simulink model "Senorless"  (R2023a)
settings: Solver=FixedStepDiscrete  StartTime=0.0  StopTime=5  FixedStep=1/FOC_FRQ  RelTol=1e-3
values from neighbouring files (symbols this model uses):
  ADC_REF = 3.6    [Senorless.sldd]
  ADC_SAMPLE_MAX = 32767.0    [Senorless.sldd]
  AMP_GAIN = 16.0    [Senorless.sldd]
  CURR_INPUT = 3276.0    [Senorless.sldd]
  CURR_KI = 380.0    [Senorless.sldd]
  CURR_KP = 0.04    [Senorless.sldd]
  CURR_LIMIT = 0.95    [Senorless.sldd]
  CURR_OVER = 6.0    [Senorless.sldd]
  CURR_POINT_GAIN = 7.0    [Senorless.sldd]
  CURR_STEP = 32760.0    [Senorless.sldd]
  CURR_UNDER = 0.03    [Senorless.sldd]
  CURR_WIDTH = 6552.0    [Senorless.sldd]
  FOC_FRQ = 25000.0    [Senorless.sldd]
  GAMMA = 32767.0    [Senorless.sldd]
  IMAX = 10.0    [Senorless.sldd]
  LPF_FRQ = 2000.0    [Senorless.sldd]
  MOTOR_DAMPER = 2.06E-7    [Senorless.sldd]
  MOTOR_FLUX = 0.00212352    [Senorless.sldd]
  MOTOR_INERTIA = 4.0E-7    [Senorless.sldd]
  MOTOR_LS = 0.000536    [Senorless.sldd]
  MOTOR_PN = 7.0    [Senorless.sldd]
  MOTOR_RS = 4.0    [Senorless.sldd]
  OPEN_IQ = 0.28    [Senorless.sldd]
  OPEN_IQ_MIN = 0.05    [Senorless.sldd]
  OPEN_IQ_SLOW = 0.1    [Senorless.sldd]
  OPEN_SPD = 1000.0    [Senorless.sldd]
  OPEN_SPD_SLOW = 180.0    [Senorless.sldd]
  OPEN_TIME = 0.5    [Senorless.sldd]
  OPEN_TIME_NFO = 0.5    [Senorless.sldd]
  PLL_LIMIT = 0.9    [Senorless.sldd]
  PLL_WIDTH = 800.0    [Senorless.sldd]
  PWM_FRQ = 96000000.0    [Senorless.sldd]
  RS_HUNT = 0.02    [Senorless.sldd]
  SMOK_FRQ = 600.0    [Senorless.sldd]
  SPD_LIMIT = 0.9    [Senorless.sldd]
  SPD_LPF_LEVEL = 0.0    [Senorless.sldd]
  SPD_MAX = 12000.0    [Senorless.sldd]
  SPD_MIN = 4000.0    [Senorless.sldd]
  SPD_REDUCE = 380.0    [Senorless.sldd]
  SPD_STEP = 6.0    [Senorless.sldd]
  SPD_WIDTH = 20.0    [Senorless.sldd]
  THETA_ERR_LIMIT = 8192.0    [Senorless.sldd]
  TS_POINT_GAIN = 10.0    [Senorless.sldd]
  UDC = 48.0    [Senorless.sldd]
  UDC_GAIN = 21.0    [Senorless.sldd]
  UDC_POINT_GAIN = 10.0    [Senorless.sldd]
undefined symbols (not defined in the file or in its folder): curr_q_ki, curr_q_kp, DiscIntNeverNeededParam, magnitude, PLL_LPF_LEVEL, Udc
libraries: simulink x20, slpidlib x5, mcbcontrolslib x2, mcbplantlib x1, autolibpmsmexterior x1, spspowerguiLib x1
(part 8 of 8)

== matlab function Senorless/FOC_PointModel/慢速开环/FreqGenerator_point2/MATLAB Function1 ==
  data: u input; y output; K_fixed input; freq_kHz input; resetTrig input; resetValue input; lowerLimit input; upperLimit input
function y = edgeTri_fixedPointIntegrator(u, K_fixed, freq_kHz, resetTrig, resetValue, lowerLimit, upperLimit)
% fixedPointIntegrator - 定点积分器（频率输入 + 复位 + 限幅 + 初始值）
%
% 输入参数说明：
%   u           - 当前输入信号（int32）
%   K_fixed     - 积分增益（已放大后的定点值，int32）
%   freq_kHz    - 控制频率（单位：kHz，如 20 表示 20kHz）
%   resetTrig   - 复位触发信号（uint8，边沿触发复位）
%   resetValue  - 复位时的初始值（int64）
%   lowerLimit  - 输出最小值（int64）
%   upperLimit  - 输出最大值（int64）
%
% 输出：
%   y           - 当前积分输出（int64）

    % 用于检测上升沿
    persistent lastResetState;
    if isempty(lastResetState)
        lastResetState = uint8(1);
    end

    % 状态变量
    persistent integratorState;
    if isempty(integratorState)
        integratorState = int64(0);
    end

    % 检测是否发生边沿触发（上升沿 或 下降沿）
    edgeTriggered = (resetTrig ~= lastResetState);

    % 如果有边沿，则复位积分器
    if edgeTriggered
        integratorState = resetValue;
    else
        % 计算 Ts（单位：μs），即 Ts = 1_000_000 / (freq_kHz * 1000)
        Ts_us = int32(1000 / freq_kHz);  % 精确到 μs（微秒）

        % 计算积分增量：delta = (K_fixed * u * Ts_us) / 1_000_000
        delta = (int64(K_fixed) * int64(u) * int64(Ts_us)) / 1000000;

        % 更新积分状态
        integratorState = integratorState + delta;

        % 饱和处理
        if integratorState > upperLimit
            integratorState = upperLimit;
        elseif integratorState < lowerLimit
            integratorState = lowerLimit;
        end
    end

    % 更新复位信号历史状态
    lastResetState = resetTrig;

    % 输出当前积分结果
    y = integratorState;
end

== matlab function Senorless/FOC_PointModel/观测器闭环//速度环/积分器//上升沿初始化/MATLAB Function ==
  data: in input; out output; n input
function out = int_shift(in,n)

out = bitshift(in,-n);

== matlab function Senorless/FOC_PointModel/Observers/Subsystem/Sin_512 ==
  data: cos_val output; angle_i16 input; sin_val output
function [cos_val, sin_val] = trig512_lookup_int16(angle_i16)
% trig512_lookup_int16 - 使用512点正弦表实现 sin 和 cos 查表（纯整数运算）
%
% 输入:
%   angle_i16 - int16 类型，范围 [-32768, 32767]
%              表示 -π ~ π（或 -180° ~ 179.9°）
% 输出:
%   sin_val   - int16 类型，正弦值范围 [-32768, 32767]
%   cos_val   - int16 类型，余弦值范围 [-32768, 32767]

    %#codegen

    % 获取正弦表（int16 类型，512 点）
    coder.const('get_sine_table_512pt');
    persistent sin512;
    if isempty(sin512)
        sin512 = get_sine_table_512pt();  % 返回 int16 类型的 512 点表
    end

    % 计算索引：将 [-32768, 32767] 映射到 [0, 511]
    index = bitand(bitshift(angle_i16, -7), 511);  % 右移 7 位并取模 512

    % 获取 sin 值（MATLAB 表从 1 开始）
    sin_val = int16(sin512(index + 1));

    % 获取 cos 值: cos(x) = sin(x + 90°) = sin(x + 128 in 512点表)
    cos_index = bitand(int32(index) + 128, 511);  % 快速取模
    cos_val = int16(sin512(cos_index + 1));
end

% =============================
% 512点正弦表定义（int16类型）
% =============================
function sin_table = get_sine_table_512pt()
    sin_table = int16([
 0 ,   402 ,   804 ,  1207 ,  1609 , ...
      2011 ,  2412 ,  2814 ,  3214 ,  3615 , ...
      4015 ,  4414 ,  4812 ,  5210 ,  5607 , ...
      6003 ,  6398 ,  6793 ,  7186 ,  7578 , ...
      7969 ,  8359 ,  8747 ,  9135 ,  9521 , ...
      9905 , 10288 , 10669 , 11049 , 11427 , ...
     11804 , 12178 , 12551 , 12922 , 13291 , ...
     13658 , 14022 , 14385 , 14746 , 15104 , ...
     15460 , 15814 , 16165 , 16514 , 16860 , ...
     17204 , 17546 , 17884 , 18220 , 18553 , ...
     18884 , 19211 , 19536 , 19857 , 20176 , ...
     20492 , 20804 , 21114 , 21420 , 21723 , ...
     22023 , 22319 , 22612 , 22902 , 23188 , ...
     23470 , 23750 , 24025 , 24297 , 24565 , ...
     24830 , 25090 , 25347 , 25601 , 25850 , ...
     26095 , 26337 , 26574 , 26808 , 27037 , ...
     27263 , 27484 , 27701 , 27914 , 28123 , ...
     28327 , 28527 , 28723 , 28915 , 29102 , ...
     29285 , 29463 , 29637 , 29806 , 29971 , ...
     30132 , 30288 , 30439 , 30586 , 30728 , ...
     30865 , 30998 , 31126 , 31250 , 31368 , ...
     31482 , 31592 , 31696 , 31796 , 31891 , ...
     31981 , 32066 , 32146 , 32222 , 32293 , ...
     32359 , 32419 , 32476 , 32527 , 32573 , ...
     32614 , 32651 , 32682 , 32709 , 32730 , ...
     32747 , 32759 , 32766 , 32767 , 32764 , ...
     32756 , 32743 , 32725 , 32703 , 32675 , ...
     32642 , 32604 , 32562 , 32514 , 32462 , ...
     32405 , 32343 , 32275 , 32204 , 32127 , ...
     32045 , 31959 , 31867 , 31771 , 31670 , ...
     31565 , 31454 , 31339 , 31219 , 31095 , ...
     30965 , 30831 , 30693 , 30549 , 30402 , ...
     30249 , 30092 , 29930 , 29764 , 29594 , ...
     29419 , 29239 , 29055 , 28867 , 28674 , ...
     28478 , 28276 , 28071 , 27861 , 27647 , ...
     27429 , 27207 , 26980 , 26750 , 26515 , ...
     26277 , 26034 , 25788 , 25538 , 25284 , ...
     25026 , 24764 , 24498 , 24229 , 23956 , ...
     23680 , 23400 , 23117 , 22830 , 22539 , ...
     22245 , 21948 , 21647 , 21344 , 21037 , ...
     20726 , 20413 , 20097 , 19777 , 19455 , ...
     19130 , 18801 , 18470 , 18136 , 17800 , ...
     17461 , 17119 , 16774 , 16427 , 16078 , ...
     15726 , 15371 , 15015 , 14656 , 14295 , ...
     13931 , 13566 , 13199 , 12829 , 12458 , ...
     12085 , 11710 , 11333 , 10954 , 10574 , ...
     10192 ,  9809 ,  9424 ,  9038 ,  8650 , ...
      8262 ,  7871 ,  7480 ,  7088 ,  6694 , ...
      6300 ,  5904 ,  5508 ,  5111 ,  4713 , ...
      4314 ,  3915 ,  3515 ,  3114 ,  2713 , ...
      2312 ,  1910 ,  1508 ,  1106 ,   704 , ...
       301 ,  -100 ,  -503 ,  -905 , -1307 , ...
     -1709 , -2111 , -2513 , -2914 , -3315 , ...
     -3715 , -4114 , -4513 , -4912 , -5309 , ...
     -5706 , -6102 , -6497 , -6891 , -7284 , ...
     -7676 , -8067 , -8456 , -8844 , -9231 , ...
     -9617 ,-10001 ,-10383 ,-10764 ,-11144 , ...
    -11521 ,-11897 ,-12271 ,-12644 ,-13014 , ...
    -13383 ,-13749 ,-14113 ,-14475 ,-14835 , ...
    -15193 ,-15549 ,-15902 ,-16253 ,-16601 , ...
    -16947 ,-17290 ,-17630 ,-17968 ,-18304 , ...
    -18636 ,-18966 ,-19293 ,-19616 ,-19937 , ...
    -20255 ,-20570 ,-20882 ,-21191 ,-21496 , ...
    -21798 ,-22097 ,-22393 ,-22685 ,-22973 , ...
    -23259 ,-23541 ,-23819 ,-24093 ,-24364 , ...
    -24632 ,-24895 ,-25155 ,-25411 ,-25663 , ...
    -25912 ,-26156 ,-26397 ,-26633 ,-26866 , ...
    -27094 ,-27318 ,-27538 ,-27755 ,-27966 , ...
    -28174 ,-28377 ,-28577 ,-28771 ,-28962 , ...
    -29148 ,-29330 ,-29507 ,-29680 ,-29848 , ...
    -30012 ,-30171 ,-30326 ,-30476 ,-30622 , ...
    -30763 ,-30899 ,-31031 ,-31157 ,-31280 , ...
    -31397 ,-31510 ,-31618 ,-31721 ,-31820 , ...
    -31914 ,-32003 ,-32087 ,-32166 ,-32240 , ...
    -32310 ,-32374 ,-32434 ,-32489 ,-32539 , ...
    -32584 ,-32624 ,-32659 ,-32689 ,-32715 , ...
    -32735 ,-32750 ,-32761 ,-32767 ,-32767 , ...
    -32763 ,-32754 ,-32739 ,-32720 ,-32696 , ...
    -32667 ,-32633 ,-32594 ,-32550 ,-32502 , ...
    -32448 ,-32390 ,-32326 ,-32258 ,-32185 , ...
    -32107 ,-32024 ,-31936 ,-31844 ,-31747 , ...
    -31644 ,-31538 ,-31426 ,-31310 ,-31189 , ...
    -31063 ,-30932 ,-30797 ,-30657 ,-30513 , ...
    -30364 ,-30210 ,-30052 ,-29889 ,-29722 , ...
    -29550 ,-29374 ,-29194 ,-29009 ,-28819 , ...
    -28626 ,-28428 ,-28225 ,-28019 ,-27808 , ...
    -27593 ,-27374 ,-27150 ,-26923 ,-26692 , ...
    -26456 ,-26217 ,-25973 ,-25726 ,-25475 , ...
    -25219 ,-24961 ,-24698 ,-24432 ,-24161 , ...
    -23888 ,-23610 ,-23330 ,-23045 ,-22757 , ...
    -22466 ,-22171 ,-21873 ,-21572 ,-21267 , ...
    -20959 ,-20648 ,-20334 ,-20017 ,-19697 , ...
    -19374 ,-19048 ,-18719 ,-18387 ,-18052 , ...
    -17715 ,-17375 ,-17033 ,-16688 ,-16340 , ...
    -15990 ,-15637 ,-15282 ,-14925 ,-14566 , ...
    -14204 ,-13840 ,-13474 ,-13106 ,-12737 , ...
    -12365 ,-11991 ,-11616 ,-11238 ,-10859 , ...
    -10479 ,-10097 , -9713 , -9328 , -8941 , ...
     -8553 , -8164 , -7774 , -7382 , -6989 , ...
     -6596 , -6201 , -5805 , -5409 , -5011 , ...
     -4613 , -4214 , -3815 , -3415 , -3014 , ...
     -2613 , -2212 , -1810 , -1408 , -1006 , ...
      -603 ,  -201 ...
    ]);
end

== matlab function Senorless/FOC_PointModel/Observers/atan_1 ==
  data: quotient input; angle_u16 output
function angle_u16  = atan(quotient)
%#codegen
%
% 使用查表法计算 arctangent (atan)
% 输入:
%   quotient - int32, 整数商 (范围应限制在 0 到 255 之间以获得最佳精度,
%                    或者其低 8 位将被用作索引)
% 输出:
%   angle_u16 - uint16, 对应的角度补偿值 (0 到 pi/2 弧度映射到 0 到 16384)

% --- 预计算的 atan 查找表 ---
% 表大小: 256 点
% 覆盖角度范围: [0, pi/2] 弧度
% 角度值映射: [0, pi/2] -> [0, 16384] (uint16)
persistent atan256;
if isempty(atan256)
    atan256 = get_atan_table_256pt();
end

% --- 主处理逻辑 ---

% 处理负输入
% if quotient < int32(0)
%     angle_u16 = uint16(0);
%     index = int32(0);
%     return;
% end

% --- 查表逻辑 ---
index = quotient;
if quotient < 0
    index = -quotient;
end

% 边界检查
if index < int32(0)
    index = int32(0);
elseif index > int32(255)
    index = int32(255);
end

% MATLAB 索引从 1 开始
lut_index = index + int32(1);
% 查表并返回结果
    angle_u16 = atan256(lut_index);
end

% =============================
% 256点反正切表定义（uint16类型）
% =============================
function atan_table = get_atan_table_256pt()
        atan_table = uint16([...
        0, 64, 128, 192, 256, 320, 384, 448, 512, 576, 640, 704, 768, 832, 896, 960, ...
        1024, 1088, 1152, 1216, 1280, 1344, 1408, 1472, 1536, 1600, 1664, 1728, 1792, 1856, 1920, 1984, ...
        2048, 2112, 2176, 2240, 2304, 2368, 2432, 2496, 2560, 2624, 2688, 2752, 2816, 2880, 2944, 3008, ...
        3072, 3136, 3200, 3264, 3328, 3392, 3456, 3520, 3584, 3648, 3712, 3776, 3840, 3904, 3968, 4032, ...
        4096, 4160, 4224, 4288, 4352, 4416, 4480, 4544, 4608, 4672, 4736, 4800, 4864, 4928, 4992, 5056, ...
        5120, 5184, 5248, 5312, 5376, 5440, 5504, 5568, 5632, 5696, 5760, 5824, 5888, 5952, 6016, 6080, ...
        6144, 6208, 6272, 6336, 6400, 6464, 6528, 6592, 6656, 6720, 6784, 6848, 6912, 6976, 7040, 7104, ...
        7168, 7232, 7296, 7360, 7424, 7488, 7552, 7616, 7680, 7744, 7808, 7872, 7936, 8000, 8064, 8128, ...
        8192, 8256, 8320, 8384, 8448, 8512, 8576, 8640, 8704, 8768, 8832, 8896, 8960, 9024, 9088, 9152, ...
        9216, 9280, 9344, 9408, 9472, 9536, 9600, 9664, 9728, 9792, 9856, 9920, 9984, 10048, 10112, 10176, ...
        10240, 10304, 10368, 10432, 10496, 10560, 10624, 10688, 10752, 10816, 10880, 10944, 11008, 11072, 11136, 11200, ...
        11264, 11328, 11392, 11456, 11520, 11584, 11648, 11712, 11776, 11840, 11904, 11968, 12032, 12096, 12160, 12224, ...
        12288, 12352, 12416, 12480, 12544, 12608, 12672, 12736, 12800, 12864, 12928, 12992, 13056, 13120, 13184, 13248, ...
        13312, 13376, 13440, 13504, 13568, 13632, 13696, 13760, 13824, 13888, 13952, 14016, 14080, 14144, 14208, 14272, ...
        14336, 14400, 14464, 14528, 14592, 14656, 14720, 14784, 14848, 14912, 14976, 15040, 15104, 15168, 15232, 15296, ...
        15360, 15424, 15488, 15552, 15616, 15680, 15744, 15808, 15872, 15936, 16000, 16064, 16128, 16192, 16256, 16320]);
end

== matlab function Senorless/FOC_PointModel/idq_Controller/PI Controller2/MATLAB Function ==
  data: in input; out output; up input; low input
function out = Limit(in,up,low)

if(in >= up)
    in = up;
end
if(in<= low)
    in = low;
end
out = in;
end

== matlab function Senorless/FOC_PointModel/idq_Controller/PI Controller2/积分器//双边沿初始化/MATLAB Function ==
  data: in input; out output; up input; low input
function out = Limit(in,up,low)

if(in >= up)
    in = up;
end
if(in<= low)
    in = low;
end
out = in;
end

== matlab function Senorless/FOC_PointModel/idq_Controller/PI Controller2/积分器//双边沿初始化/MATLAB Function1 ==
  data: in input; out output; up input; low input
function out = Limit(in,up,low)

if(in >= up)
    in = up;
end
if(in<= low)
    in = low;
end
out = in;
end

== matlab function Senorless/FOC_PointModel/idq_Controller/PI Controller2/积分器//双边沿初始化/MATLAB Function2 ==
  data: in input; out output; n input
function out = int_shift(in,n)

out = bitshift(in,-n);

== matlab function Senorless/FOC_PointModel/Sin1_512 ==
  data: angle_u16 input; sin_val output; cos_val output
function [sin_val, cos_val] = trig512_lookup(angle_u16)
    % trig512_lookup - 使用512点正弦表实现 sin 和 cos 查表（纯整数运算）
    % 输入: angle_u16 - uint16 类型，范围 [0, 65535]
    % 输出: sin_val, cos_val - int16 类型，范围 [-32768, 32767]

    %#codegen

    coder.const('sin_table512');
    % 512点正弦表 (int16)
    persistent sin512;
    if isempty(sin512)
        sin512 = get_sine_table_512pt();  % 假设这个函数返回 int16 类型的 512 点表
    end

    % 计算索引：右移 7 位相当于除以 128（因为 2^7 = 128）
    index = uint16(bitshift(angle_u16, -7));  % 右移 7 位 => index in [0, 511]
    
    % 获取 sin 值
    sin_val = int16(sin512(index + 1));  % MATLAB 表从 1 开始

    % 获取 cos 值: cos(x) = sin(x + 90°) = sin(x + 128 in 512点表)
    cos_index = uint16(mod(uint32(index) + 128, 512));  % 快速取模
    cos_val = int16(sin512(cos_index + 1));  % MATLAB 表从 1 开始
end

% =============================
% 512点正弦表定义（int16类型）
% =============================
function sin_table = get_sine_table_512pt()
    sin_table = int16([
 0 ,   402 ,   804 ,  1207 ,  1609 , ...
      2011 ,  2412 ,  2814 ,  3214 ,  3615 , ...
      4015 ,  4414 ,  4812 ,  5210 ,  5607 , ...
      6003 ,  6398 ,  6793 ,  7186 ,  7578 , ...
      7969 ,  8359 ,  8747 ,  9135 ,  9521 , ...
      9905 , 10288 , 10669 , 11049 , 11427 , ...
     11804 , 12178 , 12551 , 12922 , 13291 , ...
     13658 , 14022 , 14385 , 14746 , 15104 , ...
     15460 , 15814 , 16165 , 16514 , 16860 , ...
     17204 , 17546 , 17884 , 18220 , 18553 , ...
     18884 , 19211 , 19536 , 19857 , 20176 , ...
     20492 , 20804 , 21114 , 21420 , 21723 , ...
     22023 , 22319 , 22612 , 22902 , 23188 , ...
     23470 , 23750 , 24025 , 24297 , 24565 , ...
     24830 , 25090 , 25347 , 25601 , 25850 , ...
     26095 , 26337 , 26574 , 26808 , 27037 , ...
     27263 , 27484 , 27701 , 27914 , 28123 , ...
     28327 , 28527 , 28723 , 28915 , 29102 , ...
     29285 , 29463 , 29637 , 29806 , 29971 , ...
     30132 , 30288 , 30439 , 30586 , 30728 , ...
     30865 , 30998 , 31126 , 31250 , 31368 , ...
     31482 , 31592 , 31696 , 31796 , 31891 , ...
     31981 , 32066 , 32146 , 32222 , 32293 , ...
     32359 , 32419 , 32476 , 32527 , 32573 , ...
     32614 , 32651 , 32682 , 32709 , 32730 , ...
     32747 , 32759 , 32766 , 32767 , 32764 , ...
     32756 , 32743 , 32725 , 32703 , 32675 , ...
     32642 , 32604 , 32562 , 32514 , 32462 , ...
     32405 , 32343 , 32275 , 32204 , 32127 , ...
     32045 , 31959 , 31867 , 31771 , 31670 , ...
     31565 , 31454 , 31339 , 31219 , 31095 , ...
     30965 , 30831 , 30693 , 30549 , 30402 , ...
     30249 , 30092 , 29930 , 29764 , 29594 , ...
     29419 , 29239 , 29055 , 28867 , 28674 , ...
     28478 , 28276 , 28071 , 27861 , 27647 , ...
     27429 , 27207 , 26980 , 26750 , 26515 , ...
     26277 , 26034 , 25788 , 25538 , 25284 , ...
     25026 , 24764 , 24498 , 24229 , 23956 , ...
     23680 , 23400 , 23117 , 22830 , 22539 , ...
     22245 , 21948 , 21647 , 21344 , 21037 , ...
     20726 , 20413 , 20097 , 19777 , 19455 , ...
     19130 , 18801 , 18470 , 18136 , 17800 , ...
     17461 , 17119 , 16774 , 16427 , 16078 , ...
     15726 , 15371 , 15015 , 14656 , 14295 , ...
     13931 , 13566 , 13199 , 12829 , 12458 , ...
     12085 , 11710 , 11333 , 10954 , 10574 , ...
     10192 ,  9809 ,  9424 ,  9038 ,  8650 , ...
      8262 ,  7871 ,  7480 ,  7088 ,  6694 , ...
      6300 ,  5904 ,  5508 ,  5111 ,  4713 , ...
      4314 ,  3915 ,  3515 ,  3114 ,  2713 , ...
      2312 ,  1910 ,  1508 ,  1106 ,   704 , ...
       301 ,  -100 ,  -503 ,  -905 , -1307 , ...
     -1709 , -2111 , -2513 , -2914 , -3315 , ...
     -3715 , -4114 , -4513 , -4912 , -5309 , ...
     -5706 , -6102 , -6497 , -6891 , -7284 , ...
     -7676 , -8067 , -8456 , -8844 , -9231 , ...
     -9617 ,-10001 ,-10383 ,-10764 ,-11144 , ...
    -11521 ,-11897 ,-12271 ,-12644 ,-13014 , ...
    -13383 ,-13749 ,-14113 ,-14475 ,-14835 , ...
    -15193 ,-15549 ,-15902 ,-16253 ,-16601 , ...
    -16947 ,-17290 ,-17630 ,-17968 ,-18304 , ...
    -18636 ,-18966 ,-19293 ,-19616 ,-19937 , ...
    -20255 ,-20570 ,-20882 ,-21191 ,-21496 , ...
    -21798 ,-22097 ,-22393 ,-22685 ,-22973 , ...
    -23259 ,-23541 ,-23819 ,-24093 ,-24364 , ...
    -24632 ,-24895 ,-25155 ,-25411 ,-25663 , ...
    -25912 ,-26156 ,-26397 ,-26633 ,-26866 , ...
    -27094 ,-27318 ,-27538 ,-27755 ,-27966 , ...
    -28174 ,-28377 ,-28577 ,-28771 ,-28962 , ...
    -29148 ,-29330 ,-29507 ,-29680 ,-29848 , ...
    -30012 ,-30171 ,-30326 ,-30476 ,-30622 , ...
    -30763 ,-30899 ,-31031 ,-31157 ,-31280 , ...
    -31397 ,-31510 ,-31618 ,-31721 ,-31820 , ...
    -31914 ,-32003 ,-32087 ,-32166 ,-32240 , ...
    -32310 ,-32374 ,-32434 ,-32489 ,-32539 , ...
    -32584 ,-32624 ,-32659 ,-32689 ,-32715 , ...
    -32735 ,-32750 ,-32761 ,-32767 ,-32767 , ...
    -32763 ,-32754 ,-32739 ,-32720 ,-32696 , ...
    -32667 ,-32633 ,-32594 ,-32550 ,-32502 , ...
    -32448 ,-32390 ,-32326 ,-32258 ,-32185 , ...
    -32107 ,-32024 ,-31936 ,-31844 ,-31747 , ...
    -31644 ,-31538 ,-31426 ,-31310 ,-31189 , ...
    -31063 ,-30932 ,-30797 ,-30657 ,-30513 , ...
    -30364 ,-30210 ,-30052 ,-29889 ,-29722 , ...
    -29550 ,-29374 ,-29194 ,-29009 ,-28819 , ...
    -28626 ,-28428 ,-28225 ,-28019 ,-27808 , ...
    -27593 ,-27374 ,-27150 ,-26923 ,-26692 , ...
    -26456 ,-26217 ,-25973 ,-25726 ,-25475 , ...
    -25219 ,-24961 ,-24698 ,-24432 ,-24161 , ...
    -23888 ,-23610 ,-23330 ,-23045 ,-22757 , ...
    -22466 ,-22171 ,-21873 ,-21572 ,-21267 , ...
    -20959 ,-20648 ,-20334 ,-20017 ,-19697 , ...
    -19374 ,-19048 ,-18719 ,-18387 ,-18052 , ...
    -17715 ,-17375 ,-17033 ,-16688 ,-16340 , ...
    -15990 ,-15637 ,-15282 ,-14925 ,-14566 , ...
    -14204 ,-13840 ,-13474 ,-13106 ,-12737 , ...
    -12365 ,-11991 ,-11616 ,-11238 ,-10859 , ...
    -10479 ,-10097 , -9713 , -9328 , -8941 , ...
     -8553 , -8164 , -7774 , -7382 , -6989 , ...
     -6596 , -6201 , -5805 , -5409 , -5011 , ...
     -4613 , -4214 , -3815 , -3415 , -3014 , ...
     -2613 , -2212 , -1810 , -1408 , -1006 , ...
      -603 ,  -201 ...
    ]);
end
